simulink library "TYPEA_MASTER"  (Simulink 8.6)
settings: Solver=ode45  StartTime=0.0  StopTime=10.0  RelTol=1e-3
undefined symbols (not defined in the file): CRYP_OLSERVO, PAY_OLSERVO
libraries: cdsFilt x12, GAS_MODAL_MASTER x8, cdsEpicsBinIn x6, VIS_LIB x5, cdsEpicsOut x4, BIO_TYPEA_MASTER x3, cdsDacKill x3, ADV_BF_MASTER x2, cdsEpicsStringIn x2, TYPEA_GAS_MODAL_MASTER x2, ISC_common x2, CRYP_IM_MASTER x2
(part 1 of 2)
settings Model: Creator=controls  LastModifiedBy=controls

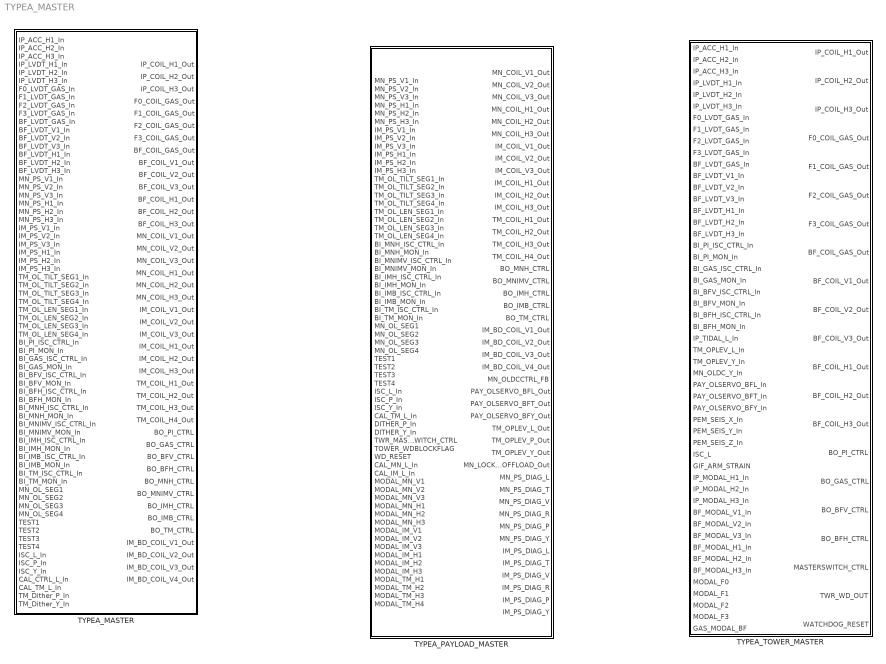
== system TYPEA_MASTER ==
  TYPEA_MASTER : Subsystem
  TYPEA_PAYLOAD_MASTER : Subsystem
  TYPEA_TOWER_MASTER : Subsystem

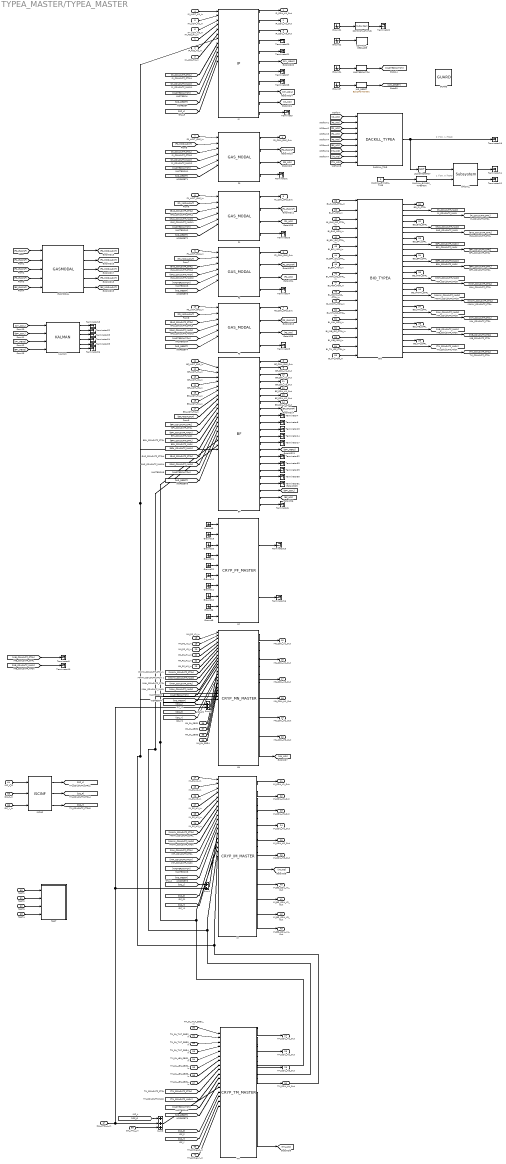
== system TYPEA_MASTER/TYPEA_MASTER ==
  note: 0 if OK, 1 if BAD
  note: 1 if OK, 0 if BAD
  IP_ACC_H1_In : Inport
  IP_ACC_H2_In : Inport  Port=2
  IP_ACC_H3_In : Inport  Port=3
  IP_LVDT_H1_In : Inport  Port=4
  IP_LVDT_H2_In : Inport  Port=5
  IP_LVDT_H3_In : Inport  Port=6
  F0_LVDT_GAS_In : Inport  Port=7
  F1_LVDT_GAS_In : Inport  Port=8
  F2_LVDT_GAS_In : Inport  Port=9
  F3_LVDT_GAS_In : Inport  Port=10
  BF_LVDT_GAS_In : Inport  Port=11
  BF_LVDT_V1_In : Inport  Port=12
  BF_LVDT_V2_In : Inport  Port=13
  BF_LVDT_V3_In : Inport  Port=14
  BF_LVDT_H1_In : Inport  Port=15
  BF_LVDT_H2_In : Inport  Port=16
  BF_LVDT_H3_In : Inport  Port=17
  MN_PS_V1_In : Inport  Port=18
  MN_PS_V2_In : Inport  Port=19
  MN_PS_V3_In : Inport  Port=20
  MN_PS_H1_In : Inport  Port=21
  MN_PS_H2_In : Inport  Port=22
  MN_PS_H3_In : Inport  Port=23
  IM_PS_V1_In : Inport  Port=24
  IM_PS_V2_In : Inport  Port=25
  IM_PS_V3_In : Inport  Port=26
  IM_PS_H1_In : Inport  Port=27
  IM_PS_H2_In : Inport  Port=28
  IM_PS_H3_In : Inport  Port=29
  TM_OL_TILT_SEG1_In : Inport  Port=30
  TM_OL_TILT_SEG2_In : Inport  Port=31
  TM_OL_TILT_SEG3_In : Inport  Port=32
  TM_OL_TILT_SEG4_In : Inport  Port=33
  TM_OL_LEN_SEG1_In : Inport  Port=34
  TM_OL_LEN_SEG2_In : Inport  Port=35
  TM_OL_LEN_SEG3_In : Inport  Port=36
  TM_OL_LEN_SEG4_In : Inport  Port=37
  BI_PI_ISC_CTRL_In : Inport  Port=38
  BI_PI_MON_In : Inport  Port=39
  BI_GAS_ISC_CTRL_In : Inport  Port=40
  BI_GAS_MON_In : Inport  Port=41
  BI_BFV_ISC_CTRL_In : Inport  Port=42
  BI_BFV_MON_In : Inport  Port=43
  BI_BFH_ISC_CTRL_In : Inport  Port=44
  BI_BFH_MON_In : Inport  Port=45
  BI_MNH_ISC_CTRL_In : Inport  Port=46
  BI_MNH_MON_In : Inport  Port=47
  BI_MNIMV_ISC_CTRL_In : Inport  Port=48
  BI_MNIMV_MON_In : Inport  Port=49
  BI_IMH_ISC_CTRL_In : Inport  Port=50
  BI_IMH_MON_In : Inport  Port=51
  BI_IMB_ISC_CTRL_In : Inport  Port=52
  BI_IMB_MON_In : Inport  Port=53
  BI_TM_ISC_CTRL_In : Inport  Port=54
  BI_TM_MON_In : Inport  Port=55
  MN_OL_SEG1 : Inport  Port=56
  MN_OL_SEG2 : Inport  Port=57
  MN_OL_SEG3 : Inport  Port=58
  MN_OL_SEG4 : Inport  Port=59
  TEST1 : Inport  Port=60
  TEST2 : Inport  Port=61
  TEST3 : Inport  Port=62
  TEST4 : Inport  Port=63
  ISC_L_In : Inport  Port=64
  ISC_P_In : Inport  Port=65
  ISC_Y_In : Inport  Port=66
  CAL_CTRL_L_In : Inport  Port=67
  CAL_TM_L_In : Inport  Port=68
  TM_Dither_P_In : Inport  Port=69
  TM_Dither_Y_In : Inport  Port=70
  BF : ADV_BF_MASTER/BF
  BIO : BIO_TYPEA_MASTER/BIO_TYPEA
  COMMISH_MESSAGE : cdsEpicsStringIn/EpicsStringIn  Tag=cdsEpicsStringIn  Description=cdsEpicsStringIn
      settings: AttributesFormatString=%<Tag>
  COMMISH_STATUS : cdsEpicsBinIn/Subsystem  Tag=cdsEpicsBinIn  Description=|
      | Purpose:                                                                            
      | Create an EPICS binary (0 or 1) input channel to the FE realtime controls.          
      |                                                                                     
      | Operation:                                                                          
      | Outputs value from an EPICS ai record. Value is binary input (bi Epics record type).
      |                                                                                     
      | Usage:                                                                              
      | Name the part with the desired EPICS channel name.
      settings: AttributesFormatString=%<Tag>
  DACKILL : cdsDacKill/Subsystem  Description=cdsDacKill
      settings: AttributesFormatString=%<Description>
  DACKILL_BYPASS_TIME : Constant  Value=0
  DACKILL_BYPASS_TIMEMON : cdsEpicsOut/Subsystem  Tag=cdsEpicsOutput  Description=|
      | Purpose:                                          
      | Output a FE signal to an EPICS channel.           
      |                                                   
      | Operation:                                        
      | Takes input value and passes it to EPICS record.  
      |                                                   
      | Usage:                                            
      | Name the part with the desired EPICS rrecord name.
      settings: AttributesFormatString=%<Tag>
  DACKILL_TRIG : VIS_LIB/DACKILL_TYPEA
  F{0..3} (4 alike) : GAS_MODAL_MASTER/GAS_MODAL
  GASMODAL : TYPEA_GAS_MODAL_MASTER/GASMODAL
  GUARD : ISC_common/GUARD
  Ground{1..2,4,6..12,19..22} (14 alike) : Ground
  IM : CRYP_IM_MASTER/CRYP_IM_MASTER  Description=SIXOSEMSTAGE_FACE_MASTER
  IP : ADV_IP_MASTER/IP
  ISCINF : VIS_LIB/ISCINF
  KALMAN : KALMAN_MASTER/KALMAN
  LogicalOperator : Logic  Operator=NOT  AllPortsSameDT=off  OutDataTypeStr=boolean
  MASTERSWITCH : cdsEpicsBinIn/Subsystem  Tag=cdsEpicsBinIn  Description=|
      | Purpose:                                                                            
      | Create an EPICS binary (0 or 1) input channel to the FE realtime controls.          
      |                                                                                     
      | Operation:                                                                          
      | Outputs value from an EPICS ai record. Value is binary input (bi Epics record type).
      |                                                                                     
      | Usage:                                                                              
      | Name the part with the desired EPICS channel name.
      settings: AttributesFormatString=%<Tag>
  MN : CRYP_MN_MASTER/CRYP_MN_MASTER  Description=SIXOSEMSTAGE_FACE_MASTER
  PF : CRYP_PF_MASTER/CRYP_PF_MASTER
  Sum1 : Sum
  Sum2 : Sum
  Sum3 : Sum  Inputs=+++
  TEST : Subsystem
  TM : CRYP_TM_MASTER/CRYP_TM_MASTER
  Terminator{,1..33} (34 alike) : Terminator
  WD_RESET : cdsEpicsMomentary/EpicsMomentary  Tag=cdsEpicsMomentary
      settings: AttributesFormatString=%<Tag>
  IP_COIL_H1_Out : Outport
  IP_COIL_H2_Out : Outport  Port=2
  IP_COIL_H3_Out : Outport  Port=3
  F0_COIL_GAS_Out : Outport  Port=4
  F1_COIL_GAS_Out : Outport  Port=5
  F2_COIL_GAS_Out : Outport  Port=6
  F3_COIL_GAS_Out : Outport  Port=7
  BF_COIL_GAS_Out : Outport  Port=8
  BF_COIL_V1_Out : Outport  Port=9
  BF_COIL_V2_Out : Outport  Port=10
  BF_COIL_V3_Out : Outport  Port=11
  BF_COIL_H1_Out : Outport  Port=12
  BF_COIL_H2_Out : Outport  Port=13
  BF_COIL_H3_Out : Outport  Port=14
  MN_COIL_V1_Out : Outport  Port=15
  MN_COIL_V2_Out : Outport  Port=16
  MN_COIL_V3_Out : Outport  Port=17
  MN_COIL_H1_Out : Outport  Port=18
  MN_COIL_H2_Out : Outport  Port=19
  MN_COIL_H3_Out : Outport  Port=20
  IM_COIL_V1_Out : Outport  Port=21
  IM_COIL_V2_Out : Outport  Port=22
  IM_COIL_V3_Out : Outport  Port=23
  IM_COIL_H1_Out : Outport  Port=24
  IM_COIL_H2_Out : Outport  Port=25
  IM_COIL_H3_Out : Outport  Port=26
  TM_COIL_H1_Out : Outport  Port=27
  TM_COIL_H2_Out : Outport  Port=28
  TM_COIL_H3_Out : Outport  Port=29
  TM_COIL_H4_Out : Outport  Port=30
  BO_PI_CTRL : Outport  Port=31
  BO_GAS_CTRL : Outport  Port=32
  BO_BFV_CTRL : Outport  Port=33
  BO_BFH_CTRL : Outport  Port=34
  BO_MNH_CTRL : Outport  Port=35
  BO_MNIMV_CTRL : Outport  Port=36
  BO_IMH_CTRL : Outport  Port=37
  BO_IMB_CTRL : Outport  Port=38
  BO_TM_CTRL : Outport  Port=39
  IM_BD_COIL_V1_Out : Outport  Port=40
  IM_BD_COIL_V2_Out : Outport  Port=41
  IM_BD_COIL_V3_Out : Outport  Port=42
  IM_BD_COIL_V4_Out : Outport  Port=43
  wires:
  IP_LVDT_H2_In/1 -> IP/2
  IP_ACC_H2_In/1 -> IP/5
  IP_LVDT_H1_In/1 -> IP/1
  IP_ACC_H1_In/1 -> IP/4
  IP_LVDT_H3_In/1 -> IP/3
  IP_ACC_H3_In/1 -> IP/6
  IP/1 -> IP_COIL_H1_Out/1
  IP/2 -> IP_COIL_H2_Out/1
  WD_RESET/1 -> [WD_RESET]
  Ground7/1 -> WD_RESET/1
  Ground4/1 -> MASTERSWITCH/1
  MASTERSWITCH/1 -> [MASTERSWITCH]
  Ground2/1 -> COMMISH_MESSAGE/1
  COMMISH_STATUS/1 -> Terminator2/1
  Ground1/1 -> COMMISH_STATUS/1
  BF_LVDT_GAS_In/1 -> BF/1
  BF_LVDT_V1_In/1 -> BF/2
  BF_LVDT_V2_In/1 -> BF/3
  BF_LVDT_H2_In/1 -> BF/6
  BF_LVDT_V3_In/1 -> BF/4
  BF_LVDT_H3_In/1 -> BF/7
  BF_LVDT_H1_In/1 -> BF/5
  [MASTERSWITCH] -> F0/5
  [WD_RESET] -> F0/6
  [MASTERSWITCH] -> F1/5
  [WD_RESET] -> F1/6
  [MASTERSWITCH] -> F2/5
  [WD_RESET] -> F2/6
  [MASTERSWITCH] -> F3/5
  [WD_RESET] -> F3/6
  [MASTERSWITCH] -> BF/15
  [WD_RESET] -> BF/16
  DACKILL_TRIG/1 -> LogicalOperator/1, Terminator19/1
  LogicalOperator/1 -> DACKILL/1
  DACKILL_BYPASS_TIMEMON/1 -> DACKILL/2
  DACKILL_BYPASS_TIME/1 -> DACKILL_BYPASS_TIMEMON/1
  DACKILL/1 -> Terminator11/1
  DACKILL/2 -> Terminator12/1
  F1/3 -> [F1_WD]
  F2/3 -> [F2_WD]
  F3/3 -> [F3_WD]
  F1/1 -> F1_COIL_GAS_Out/1
  F2/1 -> F2_COIL_GAS_Out/1
  F3/1 -> F3_COIL_GAS_Out/1
  F1/4 -> Terminator3/1
  F2/4 -> Terminator4/1
  F3/4 -> Terminator5/1
  [PI_COILOUTF_CTRL] -> F0/3
  [PI_COILOUTF_MASK] -> F0/4
  [GAS_COILOUTF_CTRL] -> F1/3
  [GAS_COILOUTF_MASK] -> F1/4
  [GAS_COILOUTF_CTRL] -> F2/3
  [GAS_COILOUTF_MASK] -> F2/4
  [GAS_COILOUTF_CTRL] -> F3/3
  [GAS_COILOUTF_MASK] -> F3/4
  [IP_WD] -> DACKILL_TRIG/1
  [F0_WD] -> DACKILL_TRIG/2
  [F1_WD] -> DACKILL_TRIG/3
  [F2_WD] -> DACKILL_TRIG/4
  [F3_WD] -> DACKILL_TRIG/5
  [BF_WD] -> DACKILL_TRIG/6
  [MN_WD] -> DACKILL_TRIG/7
  [IM_WD] -> DACKILL_TRIG/8
  [TM_WD] -> DACKILL_TRIG/9
  IM/7 -> [IM_WD]
  BI_BFV_ISC_CTRL_In/1 -> BIO/5
  BI_GAS_ISC_CTRL_In/1 -> BIO/3
  BI_BFV_MON_In/1 -> BIO/6
  BI_GAS_MON_In/1 -> BIO/4
  BI_PI_ISC_CTRL_In/1 -> BIO/1
  BI_PI_MON_In/1 -> BIO/2
  BIO/1 -> BO_PI_CTRL/1
  BIO/4 -> BO_GAS_CTRL/1
  BIO/7 -> BO_BFV_CTRL/1
  BIO/2 -> [PI_COILOUTF_MASK]
  BIO/5 -> [GAS_COILOUTF_MASK]
  BIO/8 -> [BFV_COILOUTF_MASK]
  BIO/3 -> [PI_COILOUTF_CTRL]
  BIO/6 -> [GAS_COILOUTF_CTRL]
  BIO/9 -> [BFV_COILOUTF_CTRL]
  [IMB_COILOUTF_CTRL] -> Terminator9/1
  [IMB_COILOUTF_MASK] -> Terminator10/1
  BIO/11 -> [BFH_COILOUTF_MASK]
  BIO/12 -> [BFH_COILOUTF_CTRL]
  BIO/10 -> BO_BFH_CTRL/1
  BI_BFH_ISC_CTRL_In/1 -> BIO/7
  BI_MNH_MON_In/1 -> BIO/10
  BI_MNH_ISC_CTRL_In/1 -> BIO/9
  BI_IMB_ISC_CTRL_In/1 -> BIO/15
  BI_TM_ISC_CTRL_In/1 -> BIO/17
  BI_BFH_MON_In/1 -> BIO/8
  BI_TM_MON_In/1 -> BIO/18
  BI_IMB_MON_In/1 -> BIO/16
  BIO/13 -> BO_MNH_CTRL/1
  BIO/14 -> [MNH_COILOUTF_MASK]
  BIO/15 -> [MNH_COILOUTF_CTRL]
  [BFV_COILOUTF_CTRL] -> BF/9
  [BFV_COILOUTF_MASK] -> BF/10
  [BFH_COILOUTF_CTRL] -> BF/11
  [BFH_COILOUTF_MASK] -> BF/12
  [GAS_COILOUTF_CTRL] -> BF/13
  [GAS_COILOUTF_MASK] -> BF/14
  [MASTERSWITCH] -> IM/11
  [WD_RESET] -> IM/12
  IM/1 -> IM_COIL_V1_Out/1
  IM/2 -> IM_COIL_V2_Out/1
  IM/3 -> IM_COIL_V3_Out/1
  IM/4 -> IM_COIL_H1_Out/1
  IM/5 -> IM_COIL_H2_Out/1
  [MASTERSWITCH] -> MN/11
  [WD_RESET] -> MN/12
  MN_PS_V3_In/1 -> MN/3
  MN_PS_H1_In/1 -> MN/4
  MN_PS_H2_In/1 -> MN/5
  MN_PS_H3_In/1 -> MN/6
  MN_PS_V1_In/1 -> MN/1
  MN_PS_V2_In/1 -> MN/2
  Ground19/1 -> PF/2
  Ground9/1 -> PF/1
  Ground22/1 -> PF/5
  Ground10/1 -> PF/6
  Ground21/1 -> PF/4
  Ground11/1 -> PF/7
  Ground20/1 -> PF/3
  Ground6/1 -> PF/9
  Ground12/1 -> PF/8
  Ground8/1 -> PF/10
  PF/1 -> Terminator15/1
  PF/2 -> Terminator16/1
  TM_OL_TILT_SEG1_In/1 -> TM/1
  TM_OL_LEN_SEG1_In/1 -> TM/5
  TM_OL_TILT_SEG2_In/1 -> TM/2
  TM_OL_TILT_SEG3_In/1 -> TM/3
  TM_OL_LEN_SEG4_In/1 -> TM/8
  TM_OL_TILT_SEG4_In/1 -> TM/4
  TM_OL_LEN_SEG2_In/1 -> TM/6
  TM_OL_LEN_SEG3_In/1 -> TM/7
  MN/6 -> MN_COIL_H3_Out/1
  MN/5 -> MN_COIL_H2_Out/1
  MN/4 -> MN_COIL_H1_Out/1
  MN/3 -> MN_COIL_V3_Out/1
  MN/2 -> MN_COIL_V2_Out/1
  MN/1 -> MN_COIL_V1_Out/1
  IM_PS_V3_In/1 -> IM/3
  IM_PS_H1_In/1 -> IM/4
  IM_PS_H2_In/1 -> IM/5
  IM_PS_H3_In/1 -> IM/6
  IM_PS_V1_In/1 -> IM/1
  IM_PS_V2_In/1 -> IM/2
  TM/1 -> TM_COIL_H1_Out/1
  TM/2 -> TM_COIL_H2_Out/1
  TM/3 -> TM_COIL_H3_Out/1
  TM/4 -> TM_COIL_H4_Out/1
  BIO/19 -> BO_IMH_CTRL/1
  BIO/25 -> BO_TM_CTRL/1
  BIO/22 -> BO_IMB_CTRL/1
  BIO/16 -> BO_MNIMV_CTRL/1
  BIO/17 -> [MNIMV_COILOUTF_MASK]
  BIO/26 -> [TM_COILOUTF_MASK]
  BIO/20 -> [IMH_COILOUTF_MASK]
  BIO/23 -> [IMB_COILOUTF_MASK]
  BIO/24 -> [IMB_COILOUTF_CTRL]
  BIO/18 -> [MNIMV_COILOUTF_CTRL]
  BIO/27 -> [TM_COILOUTF_CTRL]
  BIO/21 -> [IMH_COILOUTF_CTRL]
  BI_MNIMV_MON_In/1 -> BIO/12
  BI_IMH_MON_In/1 -> BIO/14
  BI_MNIMV_ISC_CTRL_In/1 -> BIO/11
  BI_IMH_ISC_CTRL_In/1 -> BIO/13
  [MNIMV_COILOUTF_CTRL] -> IM/7
  [MNIMV_COILOUTF_MASK] -> IM/8
  [IMH_COILOUTF_CTRL] -> IM/9
  [IMH_COILOUTF_MASK] -> IM/10
  [MASTERSWITCH] -> TM/11
  [TM_COILOUTF_CTRL] -> TM/9
  [TM_COILOUTF_MASK] -> TM/10
  [WD_RESET] -> TM/12
  ISC_L_In/1 -> ISCINF/1
  ISCINF/1 -> [ISC_L]
  ISCINF/2 -> [ISC_P]
  ISCINF/3 -> [ISC_Y]
  [ISC_P] -> TM/14
  [ISC_Y] -> TM/15
  [ISC_P] -> IM/14
  [ISC_Y] -> IM/15
  [ISC_L] -> Sum2/1
  [ISC_P] -> MN/14
  [ISC_Y] -> MN/15
  MN/7 -> [MN_WD]
  TM/8 -> [TM_WD]
  MN_OL_SEG4/1 -> MN/19
  MN_OL_SEG3/1 -> MN/18
  MN_OL_SEG2/1 -> MN/17
  MN_OL_SEG1/1 -> MN/16
  [MNIMV_COILOUTF_CTRL] -> MN/7
  [MNIMV_COILOUTF_MASK] -> MN/8
  [MNH_COILOUTF_CTRL] -> MN/9
  [MNH_COILOUTF_MASK] -> MN/10
  TEST1/1 -> TEST/1(TEST1_In)
  TEST2/1 -> TEST/2(TEST2_In)
  TEST3/1 -> TEST/3(TEST3_In)
  TEST4/1 -> TEST/4(TEST4_In)
  TM/5 -> BF/17, MN/20, IM/16
  TM/6 -> BF/18, MN/21, IM/17
  TM/7 -> IP/7, BF/19, MN/22, IM/18
  [WD_RESET] -> IP/11
  [MASTERSWITCH] -> IP/10
  [PI_COILOUTF_MASK] -> IP/9
  [PI_COILOUTF_CTRL] -> IP/8
  F0/1 -> F0_COIL_GAS_Out/1
  F0/4 -> Terminator1/1
  F0/3 -> [F0_WD]
  F0_LVDT_GAS_In/1 -> F0/1
  F1_LVDT_GAS_In/1 -> F1/1
  F2_LVDT_GAS_In/1 -> F2/1
  F3_LVDT_GAS_In/1 -> F3/1
  F0/2 -> [F0_GASINF]
  F1/2 -> [F1_GASINF]
  F2/2 -> [F2_GASINF]
  F3/2 -> [F3_GASINF]
  [F2_GASINF] -> GASMODAL/3
  [F3_GASINF] -> GASMODAL/4
  [F1_GASINF] -> GASMODAL/2
  [F0_GASINF] -> GASMODAL/1
  [BF_GASINF] -> GASMODAL/5
  GASMODAL/1 -> [F0_MODALOUT]
  GASMODAL/5 -> [BF_MODALOUT]
  GASMODAL/3 -> [F2_MODALOUT]
  GASMODAL/2 -> [F1_MODALOUT]
  GASMODAL/4 -> [F3_MODALOUT]
  [F0_MODALOUT] -> F0/2
  [F1_MODALOUT] -> F1/2
  [F2_MODALOUT] -> F2/2
  [F3_MODALOUT] -> F3/2
  [BF_MODALOUT] -> BF/8
  BF/1 -> BF_COIL_GAS_Out/1
  BF/2 -> BF_COIL_V1_Out/1
  BF/3 -> BF_COIL_V2_Out/1
  BF/4 -> BF_COIL_V3_Out/1
  BF/5 -> BF_COIL_H1_Out/1
  BF/6 -> BF_COIL_H2_Out/1
  BF/7 -> BF_COIL_H3_Out/1
  BF/8 -> [BF_GASINF]
  BF/9 -> Terminator7/1
  BF/10 -> Terminator8/1
  BF/11 -> Terminator13/1
  BF/12 -> Terminator14/1
  BF/13 -> Terminator17/1
  [IPY_COIL] -> KALMAN/1
  [BFY_COIL] -> KALMAN/2
  KALMAN/1 -> Terminator18/1
  KALMAN/2 -> Terminator22/1
  KALMAN/3 -> Terminator23/1
  KALMAN/4 -> Terminator24/1
  KALMAN/5 -> Terminator25/1
  KALMAN/6 -> Terminator26/1
  IP/3 -> IP_COIL_H3_Out/1
  IP/6 -> [IPY_MEAS]
  IP/7 -> Terminator27/1
  IP/8 -> Terminator28/1
  IP/9 -> [IPY_COIL]
  IP/4 -> Terminator20/1
  IP/5 -> Terminator21/1
  IP/10 -> [IP_WD]
  IP/11 -> Terminator/1
  BF/14 -> [BFY_MEAS]
  BF/22 -> Terminator6/1
  BF/21 -> [BF_WD]
  BF/15 -> Terminator32/1
  BF/16 -> Terminator33/1
  BF/18 -> Terminator30/1
  BF/19 -> Terminator31/1
  BF/17 -> Terminator29/1
  BF/20 -> [BFY_COIL]
  [BFY_MEAS] -> KALMAN/4
  [IPY_MEAS] -> KALMAN/3
  [ISC_L] -> Sum3/1
  CAL_TM_L_In/1 -> Sum3/3
  Sum3/1 -> TM/13
  ISC_P_In/1 -> ISCINF/2
  ISC_Y_In/1 -> ISCINF/3
  IM/8 -> IM_BD_COIL_V1_Out/1
  IM/9 -> IM_BD_COIL_V2_Out/1
  IM/10 -> IM_BD_COIL_V3_Out/1
  IM/11 -> IM_BD_COIL_V4_Out/1
  IM/6 -> IM_COIL_H3_Out/1
  [ISC_L] -> IP/12
  Sum1/1 -> IM/13
  [ISC_L] -> Sum1/1
  CAL_CTRL_L_In/1 -> Sum2/2, Sum1/2, Sum3/2
  Sum2/1 -> MN/13
  TM_Dither_P_In/1 -> TM/16
  TM_Dither_Y_In/1 -> TM/17

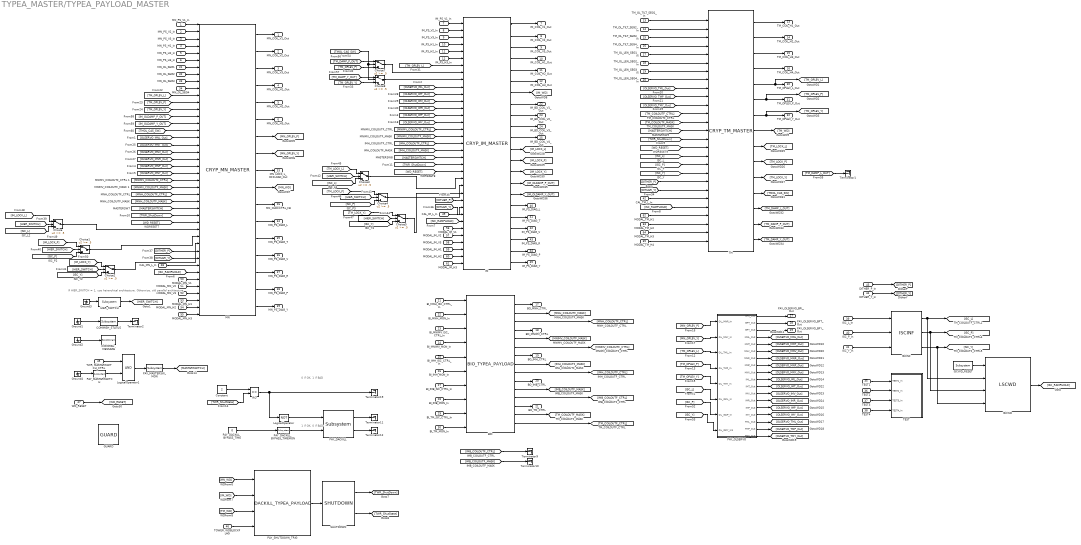
== system TYPEA_MASTER/TYPEA_PAYLOAD_MASTER ==
  note: If HIER_SWITCH = 1, use heirarchical architecture. Otherwise, old parallel architecture
  note: 0 if OK, 1 if BAD
  note: 1 if OK, 0 if BAD
  MN_PS_V1_In : Inport
  MN_PS_V2_In : Inport  Port=2
  MN_PS_V3_In : Inport  Port=3
  MN_PS_H1_In : Inport  Port=4
  MN_PS_H2_In : Inport  Port=5
  MN_PS_H3_In : Inport  Port=6
  IM_PS_V1_In : Inport  Port=7
  IM_PS_V2_In : Inport  Port=8
  IM_PS_V3_In : Inport  Port=9
  IM_PS_H1_In : Inport  Port=10
  IM_PS_H2_In : Inport  Port=11
  IM_PS_H3_In : Inport  Port=12
  TM_OL_TILT_SEG1_In : Inport  Port=13
  TM_OL_TILT_SEG2_In : Inport  Port=14
  TM_OL_TILT_SEG3_In : Inport  Port=15
  TM_OL_TILT_SEG4_In : Inport  Port=16
  TM_OL_LEN_SEG1_In : Inport  Port=17
  TM_OL_LEN_SEG2_In : Inport  Port=18
  TM_OL_LEN_SEG3_In : Inport  Port=19
  TM_OL_LEN_SEG4_In : Inport  Port=20
  BI_MNH_ISC_CTRL_In : Inport  Port=21
  BI_MNH_MON_In : Inport  Port=22
  BI_MNIMV_ISC_CTRL_In : Inport  Port=23
  BI_MNIMV_MON_In : Inport  Port=24
  BI_IMH_ISC_CTRL_In : Inport  Port=25
  BI_IMH_MON_In : Inport  Port=26
  BI_IMB_ISC_CTRL_In : Inport  Port=27
  BI_IMB_MON_In : Inport  Port=28
  BI_TM_ISC_CTRL_In : Inport  Port=29
  BI_TM_MON_In : Inport  Port=30
  MN_OL_SEG1 : Inport  Port=31
  MN_OL_SEG2 : Inport  Port=32
  MN_OL_SEG3 : Inport  Port=33
  MN_OL_SEG4 : Inport  Port=34
  TEST1 : Inport  Port=35
  TEST2 : Inport  Port=36
  TEST3 : Inport  Port=37
  TEST4 : Inport  Port=38
  ISC_L_In : Inport  Port=39
  ISC_P_In : Inport  Port=40
  ISC_Y_In : Inport  Port=41
  CAL_TM_L_In : Inport  Port=42
  DITHER_P_In : Inport  Port=43
  DITHER_Y_In : Inport  Port=44
  TWR_MASTERSWITCH_CTRL : Inport  Port=45
  TOWER_WDBLOCKFLAG : Inport  Port=46
  WD_RESET : Inport  Port=47
  CAL_MN_L_In : Inport  Port=48
  CAL_IM_L_In : Inport  Port=49
  MODAL_MN_V1 : Inport  Port=50
  MODAL_MN_V2 : Inport  Port=51
  MODAL_MN_V3 : Inport  Port=52
  MODAL_MN_H1 : Inport  Port=53
  MODAL_MN_H2 : Inport  Port=54
  MODAL_MN_H3 : Inport  Port=55
  MODAL_IM_V1 : Inport  Port=56
  MODAL_IM_V2 : Inport  Port=57
  MODAL_IM_V3 : Inport  Port=58
  MODAL_IM_H1 : Inport  Port=59
  MODAL_IM_H2 : Inport  Port=60
  MODAL_IM_H3 : Inport  Port=61
  MODAL_TM_H1 : Inport  Port=62
  MODAL_TM_H2 : Inport  Port=63
  MODAL_TM_H3 : Inport  Port=64
  MODAL_TM_H4 : Inport  Port=65
  BIO : BIO_TYPEA_MASTER/BIO_TYPEA_PAYLOAD
  COMMISH_MESSAGE : cdsEpicsStringIn/EpicsStringIn  Tag=cdsEpicsStringIn  Description=cdsEpicsStringIn
      settings: AttributesFormatString=%<Tag>
  COMMISH_STATUS : cdsEpicsBinIn/Subsystem  Tag=cdsEpicsBinIn  Description=|
      | Purpose:                                                                            
      | Create an EPICS binary (0 or 1) input channel to the FE realtime controls.          
      |                                                                                     
      | Operation:                                                                          
      | Outputs value from an EPICS ai record. Value is binary input (bi Epics record type).
      |                                                                                     
      | Usage:                                                                              
      | Name the part with the desired EPICS channel name.
      settings: AttributesFormatString=%<Tag>
  Choice{,1..5,7..8} (8 alike) : Switch  Threshold=.5
  Constant : Constant  Value=2
  GUARD : ISC_common/GUARD
  Ground{1..4} (4 alike) : Ground
  HIER_SWITCH : cdsEpicsBinIn/Subsystem  Tag=cdsEpicsBinIn  Description=|
      | Purpose:                                                                            
      | Create an EPICS binary (0 or 1) input channel to the FE realtime controls.          
      |                                                                                     
      | Operation:                                                                          
      | Outputs value from an EPICS ai record. Value is binary input (bi Epics record type).
      |                                                                                     
      | Usage:                                                                              
      | Name the part with the desired EPICS channel name.
      settings: AttributesFormatString=%<Tag>
  IM : CRYP_IM_MASTER/CRYP_IM_MASTER  Description=SIXOSEMSTAGE_FACE_MASTER
  ISCINF : VIS_LIB/ISCINF
  ISCWD : KAGRA_UTIL/LSCWD
  ISCWD_RESET : cdsEpicsIn/Subsystem  Tag=cdsEpicsIn  Description=|
      | Purpose:                                                                              
      | Create an EPICS input channel connection to the FE realtime controls.                 
      |                                                                                       
      | Operation:                                                                            
      | Outputs value from an EPICS ai record. Value is floating point with a precision of 3..
      |                                                                                       
      | Usage:                                                                                
      | Name the part with the desired EPICS channel name.
      settings: AttributesFormatString=%<Tag>
  LogicalOperator : Logic  Operator=NOT  AllPortsSameDT=off  OutDataTypeStr=boolean
  LogicalOperator1 : Logic  AllPortsSameDT=off  OutDataTypeStr=boolean
  MN : CRYP_MN_MASTER/CRYP_MN_MASTER  Description=SIXOSEMSTAGE_FACE_MASTER
  PAY_DACKILL : cdsDacKill/Subsystem  Description=cdsDacKill
      settings: AttributesFormatString=%<Description>
  PAY_DACKILL_BYPASS_TIME : Constant  Value=0
  PAY_DACKILL_BYPASS_TIMEMON : cdsEpicsOut/Subsystem  Tag=cdsEpicsOutput  Description=|
      | Purpose:                                          
      | Output a FE signal to an EPICS channel.           
      |                                                   
      | Operation:                                        
      | Takes input value and passes it to EPICS record.  
      |                                                   
      | Usage:                                            
      | Name the part with the desired EPICS rrecord name.
      settings: AttributesFormatString=%<Tag>
  PAY_MASTERSWITCH : cdsEpicsBinIn/Subsystem  Tag=cdsEpicsBinIn  Description=|
      | Purpose:                                                                            
      | Create an EPICS binary (0 or 1) input channel to the FE realtime controls.          
      |                                                                                     
      | Operation:                                                                          
      | Outputs value from an EPICS ai record. Value is binary input (bi Epics record type).
      |                                                                                     
      | Usage:                                                                              
      | Name the part with the desired EPICS channel name.
      settings: AttributesFormatString=%<Tag>
  PAY_MASTERSW_MON : cdsEpicsOut/Subsystem  Tag=cdsEpicsOutput  Description=|
      | Purpose:                                          
      | Output a FE signal to an EPICS channel.           
      |                                                   
      | Operation:                                        
      | Takes input value and passes it to EPICS record.  
      |                                                   
      | Usage:                                            
      | Name the part with the desired EPICS rrecord name.
      settings: AttributesFormatString=%<Tag>
  PAY_OLSERVO : Subsystem  AncestorBlock=CRYP_OLSERVO/PAY_OLSERVO
  PAY_SHUTDOWN_TRIG : VIS_LIB/DACKILL_TYPEA_PAYLOAD
  RO : RelationalOperator  Operator===  OutDataTypeStr=boolean
  SHUTDOWN : SHUTDOWN/SHUTDOWN
  TEST : Subsystem
  TM : CRYP_TM_MASTER/CRYP_TM_MASTER
  Terminator{1..2,9..12,19} (7 alike) : Terminator
  MN_COIL_V1_Out : Outport
  MN_COIL_V2_Out : Outport  Port=2
  MN_COIL_V3_Out : Outport  Port=3
  MN_COIL_H1_Out : Outport  Port=4
  MN_COIL_H2_Out : Outport  Port=5
  MN_COIL_H3_Out : Outport  Port=6
  IM_COIL_V1_Out : Outport  Port=7
  IM_COIL_V2_Out : Outport  Port=8
  IM_COIL_V3_Out : Outport  Port=9
  IM_COIL_H1_Out : Outport  Port=10
  IM_COIL_H2_Out : Outport  Port=11
  IM_COIL_H3_Out : Outport  Port=12
  TM_COIL_H1_Out : Outport  Port=13
  TM_COIL_H2_Out : Outport  Port=14
  TM_COIL_H3_Out : Outport  Port=15
  TM_COIL_H4_Out : Outport  Port=16
  BO_MNH_CTRL : Outport  Port=17
  BO_MNIMV_CTRL : Outport  Port=18
  BO_IMH_CTRL : Outport  Port=19
  BO_IMB_CTRL : Outport  Port=20
  BO_TM_CTRL : Outport  Port=21
  IM_BD_COIL_V1_Out : Outport  Port=22
  IM_BD_COIL_V2_Out : Outport  Port=23
  IM_BD_COIL_V3_Out : Outport  Port=24
  IM_BD_COIL_V4_Out : Outport  Port=25
  MN_OLDCCTRL_FB : Outport  Port=26
  PAY_OLSERVO_BFL_Out : Outport  Port=27
  PAY_OLSERVO_BFT_Out : Outport  Port=28
  PAY_OLSERVO_BFY_Out : Outport  Port=29
  TM_OPLEV_L_Out : Outport  Port=30
  TM_OPLEV_P_Out : Outport  Port=31
  TM_OPLEV_Y_Out : Outport  Port=32
  MN_LOCK_L_OFFLOAD_Out : Outport  Port=33
  MN_PS_DIAG_L : Outport  Port=34
  MN_PS_DIAG_T : Outport  Port=35
  MN_PS_DIAG_V : Outport  Port=36
  MN_PS_DIAG_R : Outport  Port=37
  MN_PS_DIAG_P : Outport  Port=38
  MN_PS_DIAG_Y : Outport  Port=39
  IM_PS_DIAG_L : Outport  Port=40
  IM_PS_DIAG_T : Outport  Port=41
  IM_PS_DIAG_V : Outport  Port=42
  IM_PS_DIAG_R : Outport  Port=43
  IM_PS_DIAG_P : Outport  Port=44
  IM_PS_DIAG_Y : Outport  Port=45
  wires:
  MODAL_TM_H4/1 -> TM/27
  MODAL_TM_H3/1 -> TM/26
  MODAL_TM_H2/1 -> TM/25
  MODAL_TM_H1/1 -> TM/24
  IM/19 -> IM_PS_DIAG_V/1
  IM/22 -> IM_PS_DIAG_Y/1
  IM/21 -> IM_PS_DIAG_P/1
  IM/20 -> IM_PS_DIAG_R/1
  IM/18 -> IM_PS_DIAG_T/1
  IM/17 -> IM_PS_DIAG_L/1
  MN/17 -> MN_PS_DIAG_Y/1
  MN/16 -> MN_PS_DIAG_P/1
  MN/15 -> MN_PS_DIAG_R/1
  MN/14 -> MN_PS_DIAG_V/1
  MN/13 -> MN_PS_DIAG_T/1
  MN/12 -> MN_PS_DIAG_L/1
  MODAL_IM_V3/1 -> IM/32
  MODAL_IM_H1/1 -> IM/33
  MODAL_IM_H2/1 -> IM/34
  MODAL_IM_H3/1 -> IM/35
  MODAL_IM_V1/1 -> IM/30
  MODAL_IM_V2/1 -> IM/31
  MODAL_MN_V3/1 -> MN/39
  MODAL_MN_H1/1 -> MN/40
  MODAL_MN_H2/1 -> MN/41
  MODAL_MN_H3/1 -> MN/42
  MODAL_MN_V1/1 -> MN/37
  MODAL_MN_V2/1 -> MN/38
  [ISC_RAMPHOLD] -> TM/23
  [ISC_RAMPHOLD] -> IM/29
  [ISC_RAMPHOLD] -> MN/36
  ISCWD/1 -> [ISC_RAMPHOLD]
  ISCWD_RESET/1 -> ISCWD/1
  Ground4/1 -> PAY_MASTERSWITCH/1
  PAY_MASTERSWITCH/1 -> LogicalOperator1/2
  Ground2/1 -> COMMISH_MESSAGE/1
  COMMISH_STATUS/1 -> Terminator2/1
  Ground1/1 -> COMMISH_STATUS/1
  LogicalOperator/1 -> PAY_DACKILL/1
  PAY_DACKILL_BYPASS_TIMEMON/1 -> PAY_DACKILL/2
  PAY_DACKILL_BYPASS_TIME/1 -> PAY_DACKILL_BYPASS_TIMEMON/1
  PAY_DACKILL/1 -> Terminator11/1
  PAY_DACKILL/2 -> Terminator12/1
  [MN_WD] -> PAY_SHUTDOWN_TRIG/1
  [IM_WD] -> PAY_SHUTDOWN_TRIG/2
  [TM_WD] -> PAY_SHUTDOWN_TRIG/3
  IM/7 -> [IM_WD]
  [IMB_COILOUTF_CTRL] -> Terminator9/1
  [IMB_COILOUTF_MASK] -> Terminator10/1
  BI_MNH_MON_In/1 -> BIO/2
  BI_MNH_ISC_CTRL_In/1 -> BIO/1
  BI_IMB_ISC_CTRL_In/1 -> BIO/7
  BI_TM_MON_In/1 -> BIO/10
  BI_IMB_MON_In/1 -> BIO/8
  BIO/1 -> BO_MNH_CTRL/1
  BIO/2 -> [MNH_COILOUTF_MASK]
  BIO/3 -> [MNH_COILOUTF_CTRL]
  IM/1 -> IM_COIL_V1_Out/1
  IM/2 -> IM_COIL_V2_Out/1
  IM/3 -> IM_COIL_V3_Out/1
  IM/4 -> IM_COIL_H1_Out/1
  IM/5 -> IM_COIL_H2_Out/1
  MN_PS_V3_In/1 -> MN/3
  MN_PS_H1_In/1 -> MN/4
  MN_PS_H2_In/1 -> MN/5
  MN_PS_H3_In/1 -> MN/6
  MN_PS_V1_In/1 -> MN/1
  MN_PS_V2_In/1 -> MN/2
  TM_OL_TILT_SEG1_In/1 -> TM/1
  TM_OL_LEN_SEG1_In/1 -> TM/5
  TM_OL_TILT_SEG2_In/1 -> TM/2
  TM_OL_TILT_SEG3_In/1 -> TM/3
  TM_OL_LEN_SEG4_In/1 -> TM/8
  TM_OL_TILT_SEG4_In/1 -> TM/4
  TM_OL_LEN_SEG2_In/1 -> TM/6
  TM_OL_LEN_SEG3_In/1 -> TM/7
  MN/6 -> MN_COIL_H3_Out/1
  MN/5 -> MN_COIL_H2_Out/1
  MN/4 -> MN_COIL_H1_Out/1
  MN/3 -> MN_COIL_V3_Out/1
  MN/2 -> MN_COIL_V2_Out/1
  MN/1 -> MN_COIL_V1_Out/1
  IM_PS_V3_In/1 -> IM/3
  IM_PS_H1_In/1 -> IM/4
  IM_PS_H2_In/1 -> IM/5
  IM_PS_H3_In/1 -> IM/6
  IM_PS_V1_In/1 -> IM/1
  IM_PS_V2_In/1 -> IM/2
  TM/1 -> TM_COIL_H1_Out/1
  TM/2 -> TM_COIL_H2_Out/1
  TM/3 -> TM_COIL_H3_Out/1
  TM/4 -> TM_COIL_H4_Out/1
  BIO/7 -> BO_IMH_CTRL/1
  BIO/13 -> BO_TM_CTRL/1
  BIO/10 -> BO_IMB_CTRL/1
  BIO/4 -> BO_MNIMV_CTRL/1
  BIO/5 -> [MNIMV_COILOUTF_MASK]
  BIO/14 -> [TM_COILOUTF_MASK]
  BIO/8 -> [IMH_COILOUTF_MASK]
  BIO/11 -> [IMB_COILOUTF_MASK]
  BIO/12 -> [IMB_COILOUTF_CTRL]
  BIO/6 -> [MNIMV_COILOUTF_CTRL]
  BIO/15 -> [TM_COILOUTF_CTRL]
  BIO/9 -> [IMH_COILOUTF_CTRL]
  BI_MNIMV_MON_In/1 -> BIO/4
  BI_IMH_MON_In/1 -> BIO/6
  BI_MNIMV_ISC_CTRL_In/1 -> BIO/3
  BI_IMH_ISC_CTRL_In/1 -> BIO/5
  ISC_L_In/1 -> ISCINF/1
  ISCINF/1 -> [ISC_L], ISCWD/2
  ISCINF/2 -> [ISC_P], ISCWD/3
  ISCINF/3 -> [ISC_Y], ISCWD/4
  TM/8 -> [TM_WD]
  TEST1/1 -> TEST/1(TEST1_In)
  TEST2/1 -> TEST/2(TEST2_In)
  TEST3/1 -> TEST/3(TEST3_In)
  TEST4/1 -> TEST/4(TEST4_In)
  ISC_P_In/1 -> ISCINF/2
  ISC_Y_In/1 -> ISCINF/3
  IM/8 -> IM_BD_COIL_V1_Out/1
  IM/9 -> IM_BD_COIL_V2_Out/1
  IM/10 -> IM_BD_COIL_V3_Out/1
  IM/11 -> IM_BD_COIL_V4_Out/1
  IM/6 -> IM_COIL_H3_Out/1
  BI_TM_ISC_CTRL_In/1 -> BIO/9
  TM/5 -> TM_OPLEV_L_Out/1, [TM_OPLEV_L]
  TM/6 -> TM_OPLEV_P_Out/1, [TM_OPLEV_P]
  TM/7 -> TM_OPLEV_Y_Out/1, [TM_OPLEV_Y]
  TOWER_WDBLOCKFLAG/1 -> PAY_SHUTDOWN_TRIG/4
  WD_RESET/1 -> [WD_RESET]
  PAY_SHUTDOWN_TRIG/1 -> SHUTDOWN/1
  SHUTDOWN/1 -> [TWR_ShutDown]
  SHUTDOWN/2 -> [TWR_ShutState]
  Constant/1 -> RO/1
  [TWR_ShutState] -> RO/2
  RO/1 -> Terminator19/1, LogicalOperator/1
  [TM_OPLEV_L] -> PAY_OLSERVO/3(OL_TML_In)
  [MN_OPLEV_Y] -> PAY_OLSERVO/2(OL_MNY_In)
  [TM_OPLEV_Y] -> PAY_OLSERVO/5(OL_TMY_In)
  [TM_OPLEV_P] -> PAY_OLSERVO/4(OL_TMP_In)
  [MN_OPLEV_P] -> PAY_OLSERVO/1(OL_MNP_In)
  PAY_OLSERVO/1(BFL_Out) -> PAY_OLSERVO_BFL_Out/1
  MN_OL_SEG1/1 -> MN/7
  MN_OL_SEG2/1 -> MN/8
  MN_OL_SEG3/1 -> MN/9
  MN_OL_SEG4/1 -> MN/10
  [OLSERVO_IML_Out] -> IM/10
  [OLSERVO_IMY_Out] -> IM/15
  [OLSERVO_IMP_Out] -> IM/14
  [DITHER_P] -> IM/26
  [DITHER_Y] -> IM/27
  [TWR_ShutDown] -> IM/21
  [IMH_COILOUTF_CTRL] -> IM/18
  [IMH_COILOUTF_MASK] -> IM/19
  Choice4/1 -> IM/24
  Choice5/1 -> IM/25
  [MASTERSWITCH] -> IM/20
  [MNIMV_COILOUTF_CTRL] -> IM/16
  [MNIMV_COILOUTF_MASK] -> IM/17
  [WD_RESET] -> IM/22
  Choice3/1 -> IM/23
  [OLSERVO_IMT_Out] -> IM/11
  [OLSERVO_IMV_Out] -> IM/12
  [OLSERVO_IMR_Out] -> IM/13
  MN/7 -> [MN_OPLEV_P]
  MN/8 -> [MN_OPLEV_Y]
  DITHER_P_In/1 -> [DITHER_P]
  DITHER_Y_In/1 -> [DITHER_Y]
  [OLSERVO_TMY_Out] -> TM/11
  [OLSERVO_TML_Out] -> TM/9
  [OLSERVO_TMP_Out] -> TM/10
  [MASTERSWITCH] -> TM/14
  [TM_COILOUTF_CTRL] -> TM/12
  [TM_COILOUTF_MASK] -> TM/13
  [TWR_ShutDown] -> TM/15
  [WD_RESET] -> TM/16
  [ISC_P] -> TM/18
  [ISC_Y] -> TM/19
  [ISC_L] -> TM/17
  [DITHER_Y] -> TM/21
  [DITHER_P] -> TM/20
  PAY_OLSERVO/2(BFT_Out) -> PAY_OLSERVO_BFT_Out/1
  PAY_OLSERVO/3(BFY_Out) -> PAY_OLSERVO_BFY_Out/1
  PAY_OLSERVO/16(TML_Out) -> [OLSERVO_TML_Out]
  PAY_OLSERVO/10(IML_Out) -> [OLSERVO_IML_Out]
  PAY_OLSERVO/8(MNP_Out) -> [OLSERVO_MNP_Out]
  PAY_OLSERVO/4(MNL_Out) -> [OLSERVO_MNL_Out]
  PAY_OLSERVO/5(MNT_Out) -> [OLSERVO_MNT_Out]
  PAY_OLSERVO/14(IMP_Out) -> [OLSERVO_IMP_Out]
  PAY_OLSERVO/17(TMP_Out) -> [OLSERVO_TMP_Out]
  PAY_OLSERVO/13(IMR_Out) -> [OLSERVO_IMR_Out]
  PAY_OLSERVO/18(TMY_Out) -> [OLSERVO_TMY_Out]
  PAY_OLSERVO/7(MNR_Out) -> [OLSERVO_MNR_Out]
  PAY_OLSERVO/6(MNV_Out) -> [OLSERVO_MNV_Out]
  PAY_OLSERVO/9(MNY_Out) -> [OLSERVO_MNY_Out]
  PAY_OLSERVO/11(IMT_Out) -> [OLSERVO_IMT_Out]
  PAY_OLSERVO/12(IMV_Out) -> [OLSERVO_IMV_Out]
  PAY_OLSERVO/15(IMY_Out) -> [OLSERVO_IMY_Out]
  Ground3/1 -> HIER_SWITCH/1
  HIER_SWITCH/1 -> [HIER_SWITCH]
  [HIER_SWITCH] -> Choice/2
  [ISC_L] -> Choice/3
  Choice/1 -> MN/30
  [HIER_SWITCH] -> Choice1/2
  [ISC_P] -> Choice1/3
  [HIER_SWITCH] -> Choice2/2
  [ISC_Y] -> Choice2/3
  [HIER_SWITCH] -> Choice3/2
  [ISC_L] -> Choice3/3
  [HIER_SWITCH] -> Choice4/2
  [ISC_P] -> Choice4/3
  [HIER_SWITCH] -> Choice5/2
  [ISC_Y] -> Choice5/3
  TM/9 -> [TM_LOCK_L]
  TM/10 -> [TM_LOCK_P]
  TM/11 -> [TM_LOCK_Y]
  [TM_LOCK_L] -> Choice3/1
  [TM_LOCK_P] -> Choice4/1
  [TM_LOCK_Y] -> Choice5/1
  IM/14 -> [IM_LOCK_Y]
  IM/13 -> [IM_LOCK_P]
  IM/12 -> [IM_LOCK_L]
  [IM_LOCK_Y] -> Choice2/1
  [IM_LOCK_P] -> Choice1/1
  [IM_LOCK_L] -> Choice/1
  [ISC_L] -> PAY_OLSERVO/6(OL_ISCL_In)
  [ISC_P] -> PAY_OLSERVO/7(OL_ISCP_In)
  [ISC_Y] -> PAY_OLSERVO/8(OL_ISCY_In1)
  TWR_MASTERSWITCH_CTRL/1 -> LogicalOperator1/1
  LogicalOperator1/1 -> PAY_MASTERSW_MON/1
  PAY_MASTERSW_MON/1 -> [MASTERSWITCH]
  MN/9 -> MN_LOCK_L_OFFLOAD_Out/1
  MN/10 -> [MN_WD]
  MN/11 -> MN_OLDCCTRL_FB/1
  TM/12 -> [TMOL_CAS_SW]
  TM/13 -> [TM_DAMP_L_OUT]
  TM/14 -> [TM_DAMP_P_OUT]
  TM/15 -> [TM_DAMP_Y_OUT]
  Choice8/1 -> IM/9
  Choice7/1 -> IM/8
  [TM_OPLEV_L] -> IM/7
  [TM_DAMP_L_OUT] -> Terminator1/1
  [TMOL_CAS_SW] -> Choice8/2, Choice7/2
  [TM_OPLEV_P] -> Choice7/3
  [TM_DAMP_P_OUT] -> Choice7/1
  [TM_DAMP_Y_OUT] -> Choice8/1
  [TM_OPLEV_Y] -> Choice8/3
  IM/15 -> [IM_OLDAMP_P_OUT]
  IM/16 -> [IM_OLDAMP_Y_OUT]
  [IM_OLDAMP_P_OUT] -> MN/14
  [IM_OLDAMP_Y_OUT] -> MN/15
  [TMOL_CAS_SW] -> MN/16
  [TM_OPLEV_L] -> MN/11
  [TM_OPLEV_P] -> MN/12
  [TM_OPLEV_Y] -> MN/13
  [OLSERVO_MNL_Out] -> MN/17
  [TWR_ShutDown] -> MN/28
  [OLSERVO_MNT_Out] -> MN/18
  [OLSERVO_MNV_Out] -> MN/19
  [OLSERVO_MNR_Out] -> MN/20
  [OLSERVO_MNP_Out] -> MN/21
  [OLSERVO_MNY_Out] -> MN/22
  [MASTERSWITCH] -> MN/27
  [MNH_COILOUTF_CTRL] -> MN/25
  [MNH_COILOUTF_MASK] -> MN/26
  [MNIMV_COILOUTF_CTRL] -> MN/23
  [MNIMV_COILOUTF_MASK] -> MN/24
  [WD_RESET] -> MN/29
  Choice1/1 -> MN/31
  Choice2/1 -> MN/32
  [DITHER_P] -> MN/33
  [DITHER_Y] -> MN/34
  CAL_TM_L_In/1 -> TM/22
  CAL_IM_L_In/1 -> IM/28
  CAL_MN_L_In/1 -> MN/35

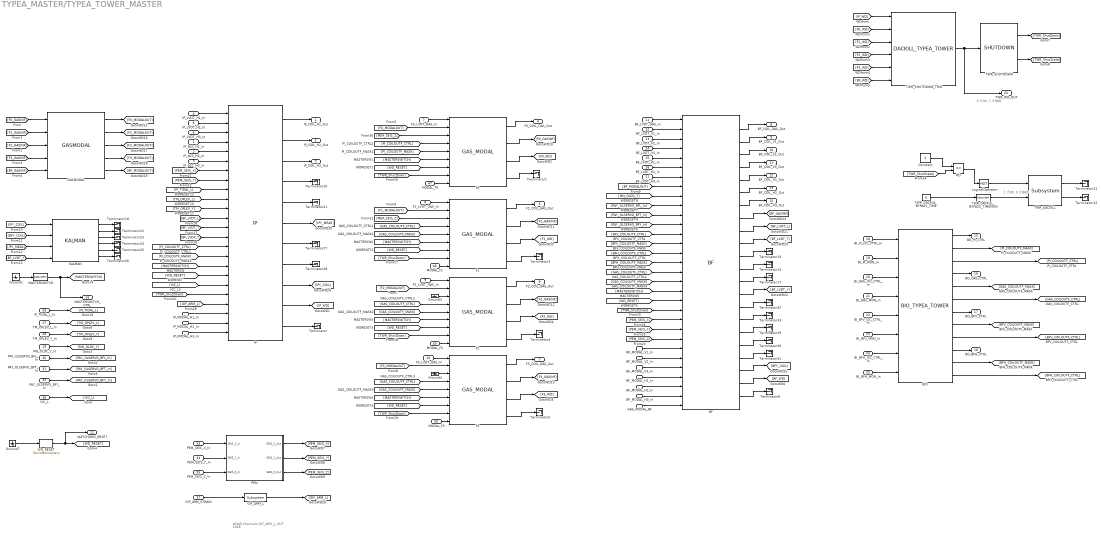
== system TYPEA_MASTER/TYPEA_TOWER_MASTER ==
  note: 1 if OK, 0 if BAD
  note: 0 if OK, 1 if BAD
  note: #DAQ Channels
      | GIF_ARM_L_OUT 2048
  IP_ACC_H1_In : Inport
  IP_ACC_H2_In : Inport  Port=2
  IP_ACC_H3_In : Inport  Port=3
  IP_LVDT_H1_In : Inport  Port=4
  IP_LVDT_H2_In : Inport  Port=5
  IP_LVDT_H3_In : Inport  Port=6
  F0_LVDT_GAS_In : Inport  Port=7
  F1_LVDT_GAS_In : Inport  Port=8
  F2_LVDT_GAS_In : Inport  Port=9
  F3_LVDT_GAS_In : Inport  Port=10
  BF_LVDT_GAS_In : Inport  Port=11
  BF_LVDT_V1_In : Inport  Port=12
  BF_LVDT_V2_In : Inport  Port=13
  BF_LVDT_V3_In : Inport  Port=14
  BF_LVDT_H1_In : Inport  Port=15
  BF_LVDT_H2_In : Inport  Port=16
  BF_LVDT_H3_In : Inport  Port=17
  BI_PI_ISC_CTRL_In : Inport  Port=18
  BI_PI_MON_In : Inport  Port=19
  BI_GAS_ISC_CTRL_In : Inport  Port=20
  BI_GAS_MON_In : Inport  Port=21
  BI_BFV_ISC_CTRL_In : Inport  Port=22
  BI_BFV_MON_In : Inport  Port=23
  BI_BFH_ISC_CTRL_In : Inport  Port=24
  BI_BFH_MON_In : Inport  Port=25
  IP_TIDAL_L_In : Inport  Port=26
  TM_OPLEV_L_In : Inport  Port=27
  TM_OPLEV_Y_In : Inport  Port=28
  MN_OLDC_Y_In : Inport  Port=29
  PAY_OLSERVO_BFL_In : Inport  Port=30
  PAY_OLSERVO_BFT_In : Inport  Port=31
  PAY_OLSERVO_BFY_In : Inport  Port=32
  PEM_SEIS_X_In : Inport  Port=33
  PEM_SEIS_Y_In : Inport  Port=34
  PEM_SEIS_Z_In : Inport  Port=35
  ISC_L : Inport  Port=36
  GIF_ARM_STRAIN : Inport  Port=37
  IP_MODAL_H1_In : Inport  Port=38
  IP_MODAL_H2_In : Inport  Port=39
  IP_MODAL_H3_In : Inport  Port=40
  BF_MODAL_V1_In : Inport  Port=41
  BF_MODAL_V2_In : Inport  Port=42
  BF_MODAL_V3_In : Inport  Port=43
  BF_MODAL_H1_In : Inport  Port=44
  BF_MODAL_H2_In : Inport  Port=45
  BF_MODAL_H3_In : Inport  Port=46
  MODAL_F0 : Inport  Port=47
  MODAL_F1 : Inport  Port=48
  MODAL_F2 : Inport  Port=49
  MODAL_F3 : Inport  Port=50
  GAS_MODAL_BF : Inport  Port=51
  BF : ADV_BF_MASTER/BF
  BIO : BIO_TYPEA_MASTER/BIO_TYPEA_TOWER
  Constant : Constant  Value=2
  F{0..3} (4 alike) : GAS_MODAL_MASTER/GAS_MODAL
  GASMODAL : TYPEA_GAS_MODAL_MASTER/GASMODAL
  GIF_ARM_L : cdsFilt/Subsystem  Tag=cdsFilt  Description=|
      | Purpose:                                                                                                                                                                                                                                  
      | Standard CDS IIR filter module.                                                                                                                                                                                                           
      |                                                                                                                                                                                                                                           
      | Operation:                                                                                                                                                                                                                                
      | Consists of 10 second order section IIR filters, plus a ramped gain stage. In FE code, also provides pre-defined test points and excitation channel inputs. The filter coefficients are defined in the LIGO system using the 'foton' tool.
      |                                                                                                                                                                                                                                           
      | Usage:                                                                                                                                                                                                                                    
      | Name the part with the desired filter module name.
      settings: AttributesFormatString=%<Tag>
  Ground{1,3..4,7} (4 alike) : Ground
  IP : ADV_IP_MASTER/IP
  KALMAN : KALMAN_MASTER/KALMAN
  LogicalOperator : Logic  Operator=NOT  AllPortsSameDT=off  OutDataTypeStr=boolean
  MASTERSWITCH : cdsEpicsBinIn/Subsystem  Tag=cdsEpicsBinIn  Description=|
      | Purpose:                                                                            
      | Create an EPICS binary (0 or 1) input channel to the FE realtime controls.          
      |                                                                                     
      | Operation:                                                                          
      | Outputs value from an EPICS ai record. Value is binary input (bi Epics record type).
      |                                                                                     
      | Usage:                                                                              
      | Name the part with the desired EPICS channel name.
      settings: AttributesFormatString=%<Tag>
  PEM : Subsystem
  RO : RelationalOperator  Operator===  OutDataTypeStr=boolean
  TWR_DACKILL : cdsDacKill/Subsystem  Description=cdsDacKill
      settings: AttributesFormatString=%<Description>
  TWR_DACKILL_BYPASS_TIME : Constant  Value=0
  TWR_DACKILL_BYPASS_TIMEMON : cdsEpicsOut/Subsystem  Tag=cdsEpicsOutput  Description=|
      | Purpose:                                          
      | Output a FE signal to an EPICS channel.           
      |                                                   
      | Operation:                                        
      | Takes input value and passes it to EPICS record.  
      |                                                   
      | Usage:                                            
      | Name the part with the desired EPICS rrecord name.
      settings: AttributesFormatString=%<Tag>
  TWR_SHUTDOWN : SHUTDOWN/SHUTDOWN
  TWR_SHUTDOWN_TRIG : VIS_LIB/DACKILL_TYPEA_TOWER
  Terminator{,1,3..6,11..14,17..18,20..33} (26 alike) : Terminator
  WD_RESET : cdsEpicsMomentary/EpicsMomentary  Tag=cdsEpicsMomentary
      settings: AttributesFormatString=%<Tag>
  IP_COIL_H1_Out : Outport
  IP_COIL_H2_Out : Outport  Port=2
  IP_COIL_H3_Out : Outport  Port=3
  F0_COIL_GAS_Out : Outport  Port=4
  F1_COIL_GAS_Out : Outport  Port=5
  F2_COIL_GAS_Out : Outport  Port=6
  F3_COIL_GAS_Out : Outport  Port=7
  BF_COIL_GAS_Out : Outport  Port=8
  BF_COIL_V1_Out : Outport  Port=9
  BF_COIL_V2_Out : Outport  Port=10
  BF_COIL_V3_Out : Outport  Port=11
  BF_COIL_H1_Out : Outport  Port=12
  BF_COIL_H2_Out : Outport  Port=13
  BF_COIL_H3_Out : Outport  Port=14
  BO_PI_CTRL : Outport  Port=15
  BO_GAS_CTRL : Outport  Port=16
  BO_BFV_CTRL : Outport  Port=17
  BO_BFH_CTRL : Outport  Port=18
  MASTERSWITCH_CTRL : Outport  Port=19
  TWR_WD_OUT : Outport  Port=20
  WATCHDOG_RESET : Outport  Port=21
  wires:
  GAS_MODAL_BF/1 -> BF/31
  MODAL_F3/1 -> F3/9
  MODAL_F2/1 -> F2/9
  MODAL_F1/1 -> F1/9
  MODAL_F0/1 -> F0/9
  IP_MODAL_H1_In/1 -> IP/22
  IP_MODAL_H2_In/1 -> IP/23
  IP_MODAL_H3_In/1 -> IP/24
  BF_MODAL_H1_In/1 -> BF/28
  BF_MODAL_H2_In/1 -> BF/29
  BF_MODAL_H3_In/1 -> BF/30
  BF_MODAL_V1_In/1 -> BF/25
  BF_MODAL_V2_In/1 -> BF/26
  BF_MODAL_V3_In/1 -> BF/27
  RO/1 -> LogicalOperator/1
  [TWR_ShutState] -> RO/2
  Constant/1 -> RO/1
  TWR_SHUTDOWN/2 -> [TWR_ShutState]
  TWR_SHUTDOWN/1 -> [TWR_ShutDown]
  TWR_SHUTDOWN_TRIG/1 -> TWR_SHUTDOWN/1, TWR_WD_OUT/1
  TWR_DACKILL/2 -> Terminator12/1
  TWR_DACKILL/1 -> Terminator11/1
  TWR_DACKILL_BYPASS_TIME/1 -> TWR_DACKILL_BYPASS_TIMEMON/1
  TWR_DACKILL_BYPASS_TIMEMON/1 -> TWR_DACKILL/2
  LogicalOperator/1 -> TWR_DACKILL/1
  WD_RESET/1 -> [WD_RESET], WATCHDOG_RESET/1
  Ground7/1 -> WD_RESET/1
  ISC_L/1 -> [ISC_L]
  MN_OLDC_Y_In/1 -> [MN_OLDC_Y]
  [IPY_MEAS] -> KALMAN/3
  [BF_LVDT_Y] -> KALMAN/4
  BF/20 -> [BFY_COIL]
  BF/17 -> Terminator29/1
  BF/19 -> Terminator31/1
  BF/18 -> Terminator30/1
  BF/16 -> Terminator33/1
  BF/15 -> Terminator32/1
  BF/21 -> [BF_WD]
  BF/14 -> [BF_LVDT_Y]
  IP/11 -> Terminator/1
  IP/10 -> [IP_WD]
  IP/5 -> Terminator21/1
  IP/4 -> Terminator20/1
  IP/9 -> [IPY_COIL]
  IP/8 -> Terminator28/1
  IP/7 -> Terminator27/1
  IP/6 -> [IPY_MEAS]
  IP/3 -> IP_COIL_H3_Out/1
  KALMAN/6 -> Terminator26/1
  KALMAN/5 -> Terminator25/1
  KALMAN/4 -> Terminator24/1
  KALMAN/3 -> Terminator23/1
  KALMAN/2 -> Terminator22/1
  KALMAN/1 -> Terminator18/1
  [BFY_COIL] -> KALMAN/2
  [IPY_COIL] -> KALMAN/1
  BF/13 -> Terminator17/1
  BF/12 -> Terminator14/1
  BF/11 -> Terminator13/1
  BF/10 -> [BF_LVDT_T]
  BF/9 -> [BF_LVDT_L]
  BF/8 -> [BF_GASINF]
  BF/7 -> BF_COIL_H3_Out/1
  BF/6 -> BF_COIL_H2_Out/1
  BF/5 -> BF_COIL_H1_Out/1
  BF/4 -> BF_COIL_V3_Out/1
  BF/3 -> BF_COIL_V2_Out/1
  BF/2 -> BF_COIL_V1_Out/1
  BF/1 -> BF_COIL_GAS_Out/1
  [BF_MODALOUT] -> BF/8
  [F3_MODALOUT] -> F3/2
  [F2_MODALOUT] -> F2/2
  [F1_MODALOUT] -> F1/2
  [F0_MODALOUT] -> F0/2
  GASMODAL/4 -> [F3_MODALOUT]
  GASMODAL/2 -> [F1_MODALOUT]
  GASMODAL/3 -> [F2_MODALOUT]
  GASMODAL/5 -> [BF_MODALOUT]
  GASMODAL/1 -> [F0_MODALOUT]
  [BF_GASINF] -> GASMODAL/5
  [F0_GASINF] -> GASMODAL/1
  [F1_GASINF] -> GASMODAL/2
  [F3_GASINF] -> GASMODAL/4
  [F2_GASINF] -> GASMODAL/3
  F3/2 -> [F3_GASINF]
  F2/2 -> [F2_GASINF]
  F1/2 -> [F1_GASINF]
  F0/2 -> [F0_GASINF]
  F3_LVDT_GAS_In/1 -> F3/1
  F2_LVDT_GAS_In/1 -> F2/1
  F1_LVDT_GAS_In/1 -> F1/1
  F0_LVDT_GAS_In/1 -> F0/1
  F0/3 -> [F0_WD]
  F0/4 -> Terminator1/1
  F0/1 -> F0_COIL_GAS_Out/1
  BI_BFH_MON_In/1 -> BIO/8
  BI_BFH_ISC_CTRL_In/1 -> BIO/7
  BIO/10 -> BO_BFH_CTRL/1
  BIO/12 -> [BFH_COILOUTF_CTRL]
  BIO/11 -> [BFH_COILOUTF_MASK]
  BIO/9 -> [BFV_COILOUTF_CTRL]
  BIO/6 -> [GAS_COILOUTF_CTRL]
  BIO/3 -> [PI_COILOUTF_CTRL]
  BIO/8 -> [BFV_COILOUTF_MASK]
  BIO/5 -> [GAS_COILOUTF_MASK]
  BIO/2 -> [PI_COILOUTF_MASK]
  BIO/7 -> BO_BFV_CTRL/1
  BIO/4 -> BO_GAS_CTRL/1
  BIO/1 -> BO_PI_CTRL/1
  BI_PI_MON_In/1 -> BIO/2
  BI_PI_ISC_CTRL_In/1 -> BIO/1
  BI_GAS_MON_In/1 -> BIO/4
  BI_BFV_MON_In/1 -> BIO/6
  BI_GAS_ISC_CTRL_In/1 -> BIO/3
  BI_BFV_ISC_CTRL_In/1 -> BIO/5
  [BF_WD] -> TWR_SHUTDOWN_TRIG/6
  [F3_WD] -> TWR_SHUTDOWN_TRIG/5
  [F2_WD] -> TWR_SHUTDOWN_TRIG/4
  [F1_WD] -> TWR_SHUTDOWN_TRIG/3
  [F0_WD] -> TWR_SHUTDOWN_TRIG/2
  [IP_WD] -> TWR_SHUTDOWN_TRIG/1
  F3/4 -> Terminator5/1
  F2/4 -> Terminator4/1
  F1/4 -> Terminator3/1
  F3/1 -> F3_COIL_GAS_Out/1
  F2/1 -> F2_COIL_GAS_Out/1
  F1/1 -> F1_COIL_GAS_Out/1
  F3/3 -> [F3_WD]
  F2/3 -> [F2_WD]
  F1/3 -> [F1_WD]
  BF_LVDT_H1_In/1 -> BF/5
  BF_LVDT_H3_In/1 -> BF/7
  BF_LVDT_V3_In/1 -> BF/4
  BF_LVDT_H2_In/1 -> BF/6
  BF_LVDT_V2_In/1 -> BF/3
  BF_LVDT_V1_In/1 -> BF/2
  BF_LVDT_GAS_In/1 -> BF/1
  MASTERSWITCH/1 -> MASTERSWITCH_CTRL/1, [MASTERSWITCH]
  IP/2 -> IP_COIL_H2_Out/1
  IP/1 -> IP_COIL_H1_Out/1
  IP_ACC_H3_In/1 -> IP/6
  IP_LVDT_H3_In/1 -> IP/3
  IP_ACC_H1_In/1 -> IP/4
  IP_LVDT_H1_In/1 -> IP/1
  IP_ACC_H2_In/1 -> IP/5
  IP_LVDT_H2_In/1 -> IP/2
  [MN_OLDC_Y] -> BF/9
  PAY_OLSERVO_BFY_In/1 -> [PAY_OLSERVO_BFY_In]
  BF/22 -> Terminator6/1
  PEM/1(SEIS_X_Out) -> [PEM_SEIS_X]
  [PEM_SEIS_X] -> IP/7
  PEM/2(SEIS_Y_Out) -> [PEM_SEIS_Y]
  PEM/3(SEIS_Z_Out) -> [PEM_SEIS_Z]
  [PEM_SEIS_Y] -> IP/8
  [PAY_OLSERVO_BFL_In] -> BF/10
  [PEM_SEIS_Y] -> BF/23
  [PEM_SEIS_X] -> BF/22
  [PAY_OLSERVO_BFT_In] -> BF/11
  [PEM_SEIS_Z] -> BF/24
  [BFH_COILOUTF_CTRL] -> BF/15
  [GAS_COILOUTF_MASK] -> BF/18
  [TWR_ShutDown] -> BF/21
  [WD_RESET] -> BF/20
  [PAY_OLSERVO_BFY_In] -> BF/12
  [MASTERSWITCH] -> BF/19
  [BFH_COILOUTF_MASK] -> BF/16
  [BFV_COILOUTF_CTRL] -> BF/13
  [GAS_COILOUTF_CTRL] -> BF/17
  [BFV_COILOUTF_MASK] -> BF/14
  PAY_OLSERVO_BFL_In/1 -> [PAY_OLSERVO_BFL_In]
  PAY_OLSERVO_BFT_In/1 -> [PAY_OLSERVO_BFT_In]
  PEM_SEIS_Y_In/1 -> PEM/2(SEIS_Y_In)
  PEM_SEIS_X_In/1 -> PEM/1(SEIS_X_In)
  PEM_SEIS_Z_In/1 -> PEM/3(SEIS_Z_In)
  TM_OPLEV_L_In/1 -> [TM_OPLEV_L]
  TM_OPLEV_Y_In/1 -> [TM_OPLEV_Y]
  GIF_ARM_L/1 -> [GIF_ARM_L]
  GIF_ARM_STRAIN/1 -> GIF_ARM_L/1
  [MASTERSWITCH] -> F0/6
  [PI_COILOUTF_CTRL] -> F0/4
  [PI_COILOUTF_MASK] -> F0/5
  [WD_RESET] -> F0/7
  [TWR_ShutDown] -> F0/8
  [GAS_COILOUTF_CTRL] -> F1/4
  [GAS_COILOUTF_MASK] -> F1/5
  [MASTERSWITCH] -> F1/6
  [WD_RESET] -> F1/7
  [TWR_ShutDown] -> F1/8
  Ground3/1 -> F2/3
  [GAS_COILOUTF_MASK] -> F2/5
  [MASTERSWITCH] -> F2/6
  [WD_RESET] -> F2/7
  [GAS_COILOUTF_CTRL] -> F2/4
  [TWR_ShutDown] -> F2/8
  Ground4/1 -> F3/3
  [GAS_COILOUTF_CTRL] -> F3/4
  [GAS_COILOUTF_MASK] -> F3/5
  [MASTERSWITCH] -> F3/6
  [WD_RESET] -> F3/7
  [TWR_ShutDown] -> F3/8
  [PEM_SEIS_Z] -> F1/3
  [PEM_SEIS_Z] -> F0/3
  Ground1/1 -> MASTERSWITCH/1
  [IP_TIDAL_L] -> IP/9
  [GIF_ARM_L] -> IP/21
  [BF_LVDT_Y] -> IP/14
  [BF_LVDT_T] -> IP/13
  [BF_LVDT_L] -> IP/12
  [TM_OPLEV_L] -> IP/10
  [TM_OPLEV_Y] -> IP/11
  [ISC_L] -> IP/19
  [MASTERSWITCH] -> IP/17
  [PI_COILOUTF_CTRL] -> IP/15
  [PI_COILOUTF_MASK] -> IP/16
  [WD_RESET] -> IP/18
  [TWR_ShutDown] -> IP/20
  IP_TIDAL_L_In/1 -> [IP_TIDAL_L]
